simulink model "PalletizeBoxesUsingCobot"  (R2024b)
settings: Solver=FixedStepDiscrete  StartTime=0.0  StopTime=Inf  FixedStep=0.01  RelTol=1e-3
PreLoadFcn:
  | rbt = exampleHelperSetUpCobot();
  | 
  | %maxNumOfBoxes = 30;
  | %boxDim = 0.2;
  | boxPosition = [-0.65 0.45 0.6];
  | 
  | % initSim.m
  | boxData = readmatrix('boxDimensions.xlsx');  % Now it's a double matrix
  | assignin('base', 'boxData', boxData);
InitFcn:
  | goal_data = readmatrix('rectangle_placements_ROT.xlsx');
StartFcn:
  | coder.extrinsic("spawnBox")
  | 
  | % Spawn the first box on the bench
  | K = [0.2, 0.2, 0.2];
  | spawnBox(0,boxPosition,K)
values from neighbouring files (symbols this model uses):
  boxDim = 0.2    [Rbt_setup.m]
  maxNumOfBoxes = 30    [Rbt_setup.m]
undefined symbols (not defined in the file or in its folder): A2, A20, I12, N2, N20, O12, O2
libraries: robotcorelib x3, robotmaniplib x3, sim3dlib x2, robotsim3dlib x1, simulink x1
settings Model: SimulationMode=accelerator  PauseTimes=1  Creator=araman  LastModifiedBy=admin
settings DebuggingCC: ReadBeforeWriteMsg=DisableAll  WriteAfterWriteMsg=DisableAll  WriteAfterReadMsg=DisableAll  MultiTaskDSMMsg=none
settings ModelReferenceCC: UpdateModelReferenceTargets=IfOutOfDate
settings SFSimCC: SFSimEcho=off

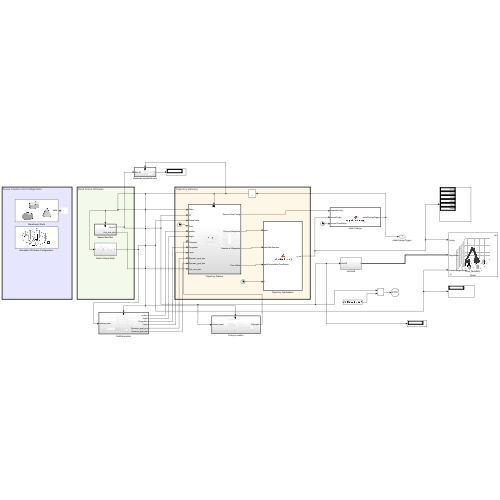
[thumbnail: Simulink's stored preview of the top-level diagram]
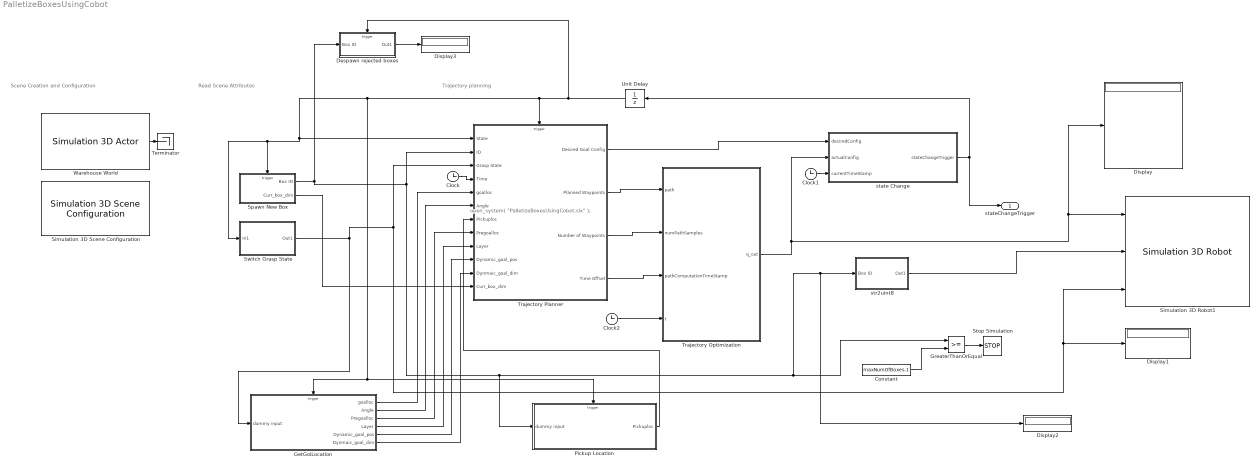
== system PalletizeBoxesUsingCobot ==
  note: open_system( "PalletizeBoxesUsingCobot.slx" );
  note: Trajectory planning
  note: Scene Creation and Configuration
  note: Read Scene Attributes
  Clock : Clock
  Clock1 : Clock
  Clock2 : Clock
  Constant : Constant  Value=maxNumOfBoxes-1
  Despawn rejected boxes : Subsystem  TreatAsAtomicUnit=on
  Display{,1..3} (4 alike) : Display
  GetGolLocation : Subsystem
  GreaterThanOrEqual : RelationalOperator  OutDataTypeStr=boolean  RndMeth=Simplest  InputSameDT=off
  Pickup Location : Subsystem  TreatAsAtomicUnit=on
  Simulation 3D Robot1 : robotsim3dlib/Simulation 3D Robot  actorInputType=RigidBodyTree Object  RigidBodyTree=rbt  ActorName=Robot  existActorChekBox=off  initialTrans=[0 0 0]  initialRot=[0 0 0]  initialConfig=[2.852 -1.623 2.216 4.223 -1.558 4.379]  EndEffector=4cup_assembly  eeOffsetInpChekBox=off  eeTargetTrans=[0 -0.2 0]  eeTargetRot=[0 0 0]  enableRegionGraspChekBox=off  regionGraspInpChekBox=off  eeTargTransDiff=[0.2 0.2 0.2]  eeTargRotDiff=[0 0 0]  inpConfEnbVal=on  inpGraspEnbVal=on  inpTransEnbVal=off  outConfEnbVal=off  outGraspEnbVal=off  outTransEnbVal=off  SampleTime=-1  ActorType=SimulinkVehicle  ID=C  aMode=6  ActorTag=Robot  Mesh=RigidBodyTree
  "Simulation 3D Scene Configuration " : sim3dlib/Simulation 3D Scene Configuration  Priority=0  ProjectFormat=Default Scenes  SceneDesc=Empty scene  ProjectName=C:\Program Files\MATLAB\R2024b\toolbox\shared\sim3d_projects\automotive_project_windows\UE\WindowsNoEditor\VehicleSimulation.exe  ScenePath=/Game/Maps/EmptyScene  EnableOpenDRIVE=off  vehTagList={'Custom';'Robot';'Scene Origin';'Warehouse'}  vehTag=Robot  FreeCameraInitialTranslation=[0, 0, 5]  FreeCameraDefaultInitialTranslation=[-6, 0, 2]  FreeCameraInitialRotation=[0, -90, 0]  FreeCameraDefaultInitialRotation=[0, -15, 0]  OpVisEn=off  Ts=0.02  EnableWindow=on  EnableRemoteAccess=off  EnableWeather=off  SunAzimuth=90  SunAltitude=40.0  EnableGeospatialSun=off  Latitude=0  Longitude=0  Date=2023-01-01  Time=10:30:00  GeoTimeZone=-5.0  SunDaylightSaving=off  wind=1  clouds=10  EnableVolumetricClouds=off  CloudCoverage=0  CloudAltitude=6  fog=0  rain=0  RaindropsEffect=off  SnowDensity=0  EnableGeospatial=off  UseTrueOrigin=off  OriginHeight=200  OriginLatitude=40.744652  OriginLongitude=-73.988864  MapStyle=Aerial  AdditionalAssetIDs=[]  UseAdvancedSunSky=off  SolarTime=11  TimeZone=-5  Day=21  Month=9  Year=2022  UseDaylightSavingTime=on  DSTStartDay=10  DSTStartMonth=3  DSTEndDay=3  DSTEndMonth=11  DSTSwitchHour=2  sensorTag=MainCamera2  sensorId=2  sensorName=MainCamera2  mountLoc=Origin  offsetFlag=off  tmountOffset=[0, 0, 0]  rmountOffset=[0, 0, 0]  HorizontalResolution=1280  VerticalResolution=720  HorizontalFOV=60  mountPoint=[0 0 0]  mountOrientation=[0 0 0]  aMode=6  ID=2  GeoTrigger=Inactive
      settings: LibrarySourceBlock=robotsim3dlib/Simulation 3D Scene Configuration
  Spawn New Box : Subsystem  TreatAsAtomicUnit=on
  Stop Simulation : Stop
  Switch Grasp State : Subsystem
  Terminator : Terminator
  Trajectory Optimization : MATLAB Function  TreatAsAtomicUnit=on
  Trajectory Planner : Subsystem
  Unit Delay : UnitDelay  InitialCondition=-1  SampleTime=-1  HasFrameUpgradeWarning=on
  Warehouse World : sim3dlib/Simulation 3D Actor  Priority=1  ActorName=Warehouse  ParentName=Scene Origin  Operation=Create at setup  InitScriptText=|  SampleTime=-1  Translation=single([0 0 0])  Rotation=single([0 0 0])  Scale=single([1 1 1])  aMode=5  ActorTag=Warehouse  ActorType=Sim3dActor  ID=2
      | Plane = sim3d.Actor(ActorName='Plane');
      | Plane.createShape('plane',[5 6 0.1]);
      | Plane.PreciseContacts = true;
      | Plane.Color = [81, 94, 120]/256;
      | add(World,Plane,Actor);
      | 
      | Base = sim3d.Actor('ActorName','collBase');
      | Base.createShape('box',[0.25,0.25,0.5]);
      | Base.Translation = [0,0.1,0.25];
      | Base.Color = [87, 67, 60]/256;
      | add(World,Base,Actor);
      | 
      | %Box spawn bench
      | Bench = sim3d.Actor('ActorName','collBench');
      | Bench.createShape('box',[0.8 0.8 0.5]);
      | Bench.Translation = [-0.5 -0.7 0.25];
      | Bench.Color = [87, 67, 60]/256;
      | add(World,Bench,Actor);
      | 
      | %Rejection conveyer
      | Bench_R = sim3d.Actor('ActorName','collBench_R');
      | Bench_R.createShape('box',[0.4 0.8 0.3]);
      | Bench_R.Translation = [-1.2 -0.7 0.25];
      | Bench_R.Color = [180, 40, 36]/256;
      | add(World,Bench_R,Actor);
      | 
      | 
      | %Layer 2 storage bench
      | Bench_2 = sim3d.Actor('ActorName','collBench_2');
      | Bench_2.createShape('box',[1.2 0.8 0.5]);
      | Bench_2.Translation = [0.4 0.8 0.25];
      | Bench_2.Color = [40, 170, 46]/256;
      | add(World,Bench_2,Actor);
      | 
      | 
      | Pallet = sim3d.Actor(ActorName='collPallet');
      | add(World,Pallet,Actor)
      | load(Pallet,"SceneAssets/PalletEuro.stl",0.001*[1 1 1]);
      | Pallet.Translation = [-1.1 -0.1 0];
  state Change : MATLAB Function  TreatAsAtomicUnit=on
  str2uint8 : Subsystem
  stateChangeTrigger : Outport
  wires:
  Warehouse World/1 -> Terminator/1
  Unit Delay/1 -> GetGolLocation/Trigger, Pickup Location/Trigger, Spawn New Box/Trigger, Switch Grasp State/1(In1), Trajectory Planner/1(State), Trajectory Planner/Trigger, Despawn rejected boxes/Trigger
  Clock/1 -> Trajectory Planner/4(Time)
  Trajectory Planner/2(Planned Waypoints) -> Trajectory Optimization/1(path)
  Trajectory Planner/3(Number of Waypoints) -> Trajectory Optimization/2(numPathSamples)
  Trajectory Planner/4(Time Offset) -> Trajectory Optimization/3(pathComputationTimeStamp)
  Trajectory Planner/1(Desired Goal Config) -> state Change/1(desiredConfig)
  Spawn New Box/1(Box ID) -> Pickup Location/1(dummy input), Display2/1, str2uint8/1(Box ID), GreaterThanOrEqual/1, Trajectory Planner/2(ID), Despawn rejected boxes/1(Box ID)
  Clock1/1 -> state Change/3(currentTimeStamp)
  state Change/1(stateChangeTrigger) -> stateChangeTrigger/1, Unit Delay/1
  Clock2/1 -> Trajectory Optimization/4(t)
  Switch Grasp State/1(Out1) -> Simulation 3D Robot1/3, Display1/1, Trajectory Planner/3(Grasp State), GetGolLocation/1(dummy input)
  Trajectory Optimization/1(q_out) -> state Change/2(actualConfig), Display/1, Simulation 3D Robot1/1
  Constant/1 -> GreaterThanOrEqual/2
  GreaterThanOrEqual/1 -> Stop Simulation/1
  GetGolLocation/1(goalloc) -> Trajectory Planner/5(goalloc)
  GetGolLocation/2(Angle) -> Trajectory Planner/6(Angle)
  str2uint8/1(Out1) -> Simulation 3D Robot1/2
  Pickup Location/1(Pickuploc) -> Trajectory Planner/7(Pickuploc)
  GetGolLocation/3(Pregoalloc) -> Trajectory Planner/8(Pregoalloc)
  GetGolLocation/4(Layer) -> Trajectory Planner/9(Layer)
  Despawn rejected boxes/1(Out1) -> Display3/1
  GetGolLocation/5(Dynamic_goal_pos) -> Trajectory Planner/10(Dynamic_goal_pos)
  GetGolLocation/6(Dynmaic_goal_dim) -> Trajectory Planner/11(Dynmaic_goal_dim)
  Spawn New Box/2(Curr_box_dim) -> Trajectory Planner/12(Curr_box_dim)

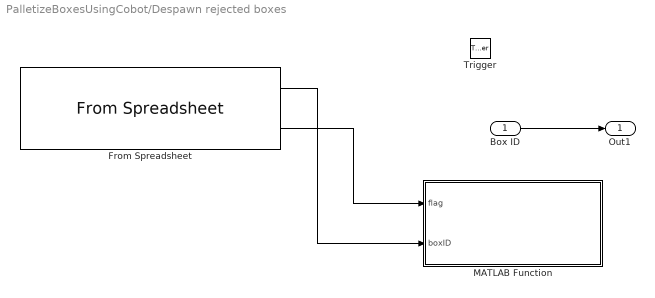
== system PalletizeBoxesUsingCobot/Despawn rejected boxes ==
  Box ID : Inport
  Trigger : TriggerPort  VariantControl=(inherit)
  From Spreadsheet : FromSpreadsheet  FileName=box_pick_goal_schedule_1.xlsx  Range=A2:A20,N2:N20  TreatFirstColumnAs=Data  SampleTime=-1
  MATLAB Function : MATLAB Function  TreatAsAtomicUnit=on
  Out1 : Outport
  wires:
  Box ID/1 -> Out1/1
  From Spreadsheet/2 -> MATLAB Function/1(flag)
  From Spreadsheet/1 -> MATLAB Function/2(boxID)

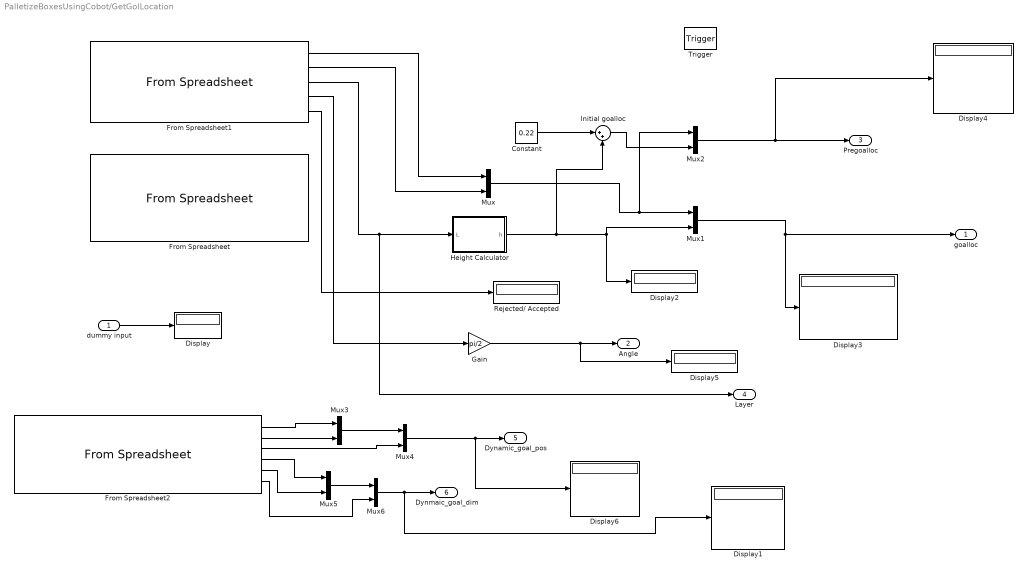
== system PalletizeBoxesUsingCobot/GetGolLocation ==
  dummy input : Inport
  Trigger : TriggerPort  VariantControl=(inherit)  PortDimensions=1
  Constant : Constant  Value=0.22
  Display{,1..6} (7 alike) : Display
  From Spreadsheet : FromSpreadsheet  FileName=test.xlsx  SheetName=Sheet3  Range=A2:B8, G2:H8, I2:I8  TreatFirstColumnAs=Data  SampleTime=-1
  From Spreadsheet1 : FromSpreadsheet  FileName=box_pick_goal_schedule_14.xlsx  SheetName=Sheet2  Range=E2:F11, K2:K11, L2:L11, N2:N11  TreatFirstColumnAs=Data  SampleTime=-1
  From Spreadsheet2 : FromSpreadsheet  FileName=box_pick_goal_schedule_14.xlsx  SheetName=Sheet3  Range=E2:I12,O2:O12  TreatFirstColumnAs=Data  SampleTime=-1
  Gain : Gain  Gain=pi/2
  Height Calculator : MATLAB Function  TreatAsAtomicUnit=on
  Initial goalloc : Sum  Inputs=|++
  Mux{,1..6} (7 alike) : Mux  Inputs=2
  Rejected/ Accepted : Display
  goalloc : Outport
  Angle : Outport  Port=2
  Pregoalloc : Outport  Port=3
  Layer : Outport  Port=4
  Dynamic_goal_pos : Outport  Port=5
  Dynmaic_goal_dim : Outport  Port=6
  wires:
  Mux/1 -> Mux1/1, Mux2/1
  dummy input/1 -> Display/1
  Mux1/1 -> Display3/1, goalloc/1
  Gain/1 -> Display5/1, Angle/1
  Height Calculator/1(h) -> Mux1/2, Display2/1, Initial goalloc/2
  Constant/1 -> Initial goalloc/1
  Initial goalloc/1 -> Mux2/2
  Mux2/1 -> Display4/1, Pregoalloc/1
  From Spreadsheet1/3 -> Layer/1, Height Calculator/1(L)
  From Spreadsheet1/2 -> Mux/2
  From Spreadsheet1/1 -> Mux/1
  From Spreadsheet1/4 -> Gain/1
  From Spreadsheet1/5 -> Rejected/ Accepted/1
  From Spreadsheet2/1 -> Mux3/1
  From Spreadsheet2/2 -> Mux3/2
  Mux3/1 -> Mux4/1
  From Spreadsheet2/3 -> Mux4/2
  From Spreadsheet2/4 -> Mux5/1
  From Spreadsheet2/5 -> Mux5/2
  Mux5/1 -> Mux6/1
  From Spreadsheet2/6 -> Mux6/2
  Mux4/1 -> Display6/1, Dynamic_goal_pos/1
  Mux6/1 -> Display1/1, Dynmaic_goal_dim/1

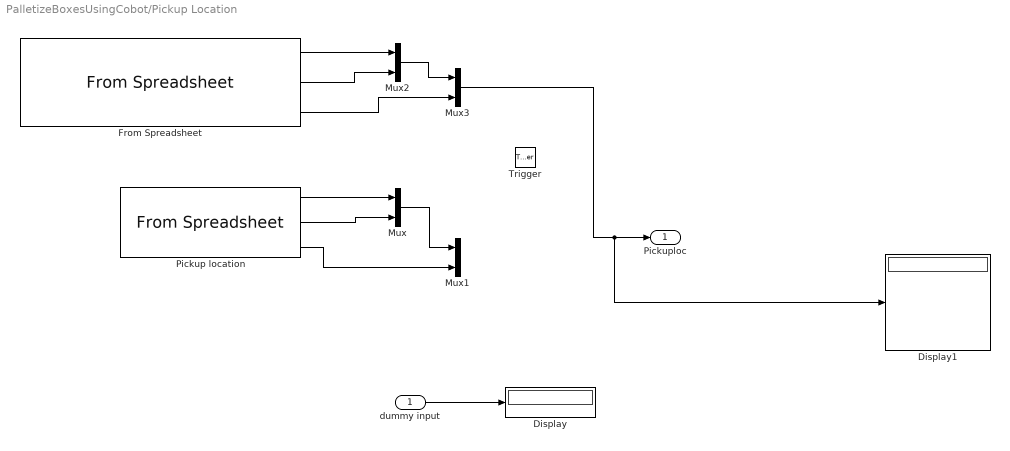
== system PalletizeBoxesUsingCobot/Pickup Location ==
  dummy input : Inport
  Trigger : TriggerPort  TriggerType=falling  VariantControl=(inherit)
  Display : Display
  Display1 : Display
  From Spreadsheet : FromSpreadsheet  FileName=box_pick_goal_schedule_14.xlsx  SheetName=Sheet2  Range=B2:D10  TreatFirstColumnAs=Data  SampleTime=-1
  Mux{,1..3} (4 alike) : Mux  Inputs=2
  Pickup location : FromSpreadsheet  FileName=test.xlsx  SheetName=Sheet3  Range=J2:L8  TreatFirstColumnAs=Data  SampleTime=-1
  Pickuploc : Outport
  wires:
  Pickup location/1 -> Mux/1
  Pickup location/2 -> Mux/2
  Pickup location/3 -> Mux1/2
  Mux/1 -> Mux1/1
  dummy input/1 -> Display/1
  From Spreadsheet/1 -> Mux2/1
  From Spreadsheet/2 -> Mux2/2
  Mux2/1 -> Mux3/1
  From Spreadsheet/3 -> Mux3/2
  Mux3/1 -> Display1/1, Pickuploc/1

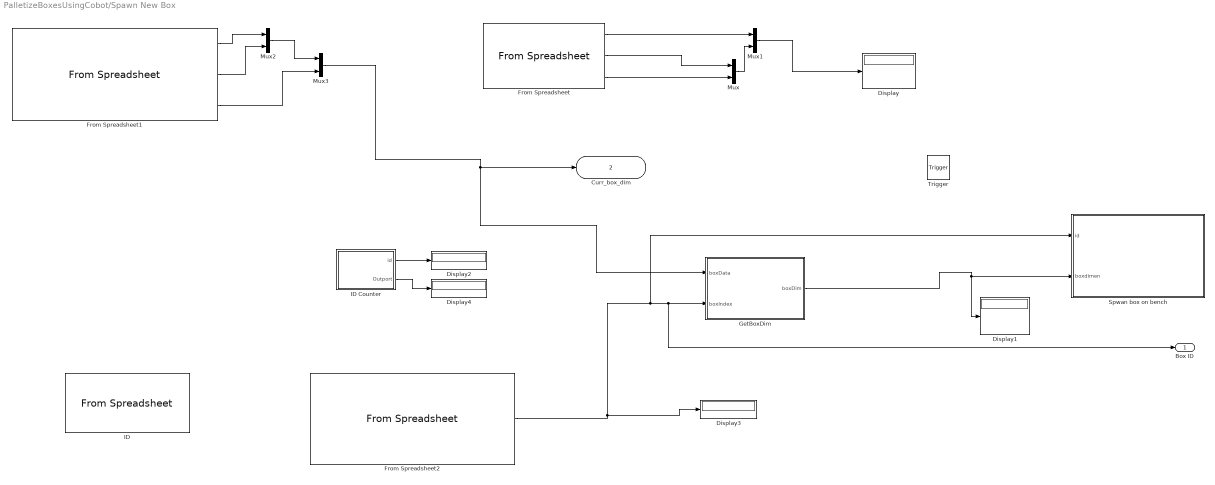
== system PalletizeBoxesUsingCobot/Spawn New Box ==
  Trigger : TriggerPort  TriggerType=falling  VariantControl=(inherit)
  Display{,1..4} (5 alike) : Display
  From Spreadsheet : FromSpreadsheet  FileName=test.xlsx  SheetName=Sheet4  Range=B2:C5, E2:E5  OutDataTypeStr=double  TreatFirstColumnAs=Data  SampleTime=-1  OutputAfterLastPoint=Ground value
  From Spreadsheet1 : FromSpreadsheet  FileName=Boxes.xlsx  SheetName=Sheet2  Range=B2:C8, E2:E8  TreatFirstColumnAs=Data  SampleTime=-1  OutputAfterLastPoint=Ground value
  From Spreadsheet2 : FromSpreadsheet  FileName=box_pick_goal_schedule_14.xlsx  SheetName=Sheet2  Range=A2:A10  TreatFirstColumnAs=Data  SampleTime=-1  OutputAfterLastPoint=Ground value
  GetBoxDim : MATLAB Function  TreatAsAtomicUnit=on
  ID : FromSpreadsheet  FileName=test.xlsx  SheetName=Sheet3  Range=N2:N8  TreatFirstColumnAs=Data  SampleTime=-1
  ID Counter : Subsystem
  Mux{,1..3} (4 alike) : Mux  Inputs=2
  Spwan box on bench : MATLAB Function  TreatAsAtomicUnit=on
  Box ID : Outport
  Curr_box_dim : Outport  Port=2
  wires:
  GetBoxDim/1(boxDim) -> Display1/1, Spwan box on bench/2(boxdimen)
  From Spreadsheet/2 -> Mux/1
  From Spreadsheet/3 -> Mux/2
  From Spreadsheet/1 -> Mux1/1
  Mux/1 -> Mux1/2
  ID Counter/1(id) -> Display2/1
  ID Counter/2(Outport) -> Display4/1
  Mux1/1 -> Display/1
  From Spreadsheet1/1 -> Mux2/1
  From Spreadsheet1/2 -> Mux2/2
  Mux2/1 -> Mux3/1
  From Spreadsheet1/3 -> Mux3/2
  Mux3/1 -> GetBoxDim/1(boxData), Curr_box_dim/1
  From Spreadsheet2/1 -> Display3/1, Spwan box on bench/1(id), Box ID/1, GetBoxDim/2(boxIndex)

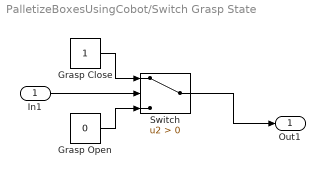
== system PalletizeBoxesUsingCobot/Switch Grasp State ==
  In1 : Inport
  Grasp Close : Constant  OutDataTypeStr=boolean
  Grasp Open : Constant  Value=0  OutDataTypeStr=boolean
  Switch : Switch  Criteria=u2 > Threshold  SaturateOnIntegerOverflow=off  InputSameDT=off
  Out1 : Outport
  wires:
  Grasp Close/1 -> Switch/1
  Switch/1 -> Out1/1
  Grasp Open/1 -> Switch/3
  In1/1 -> Switch/2

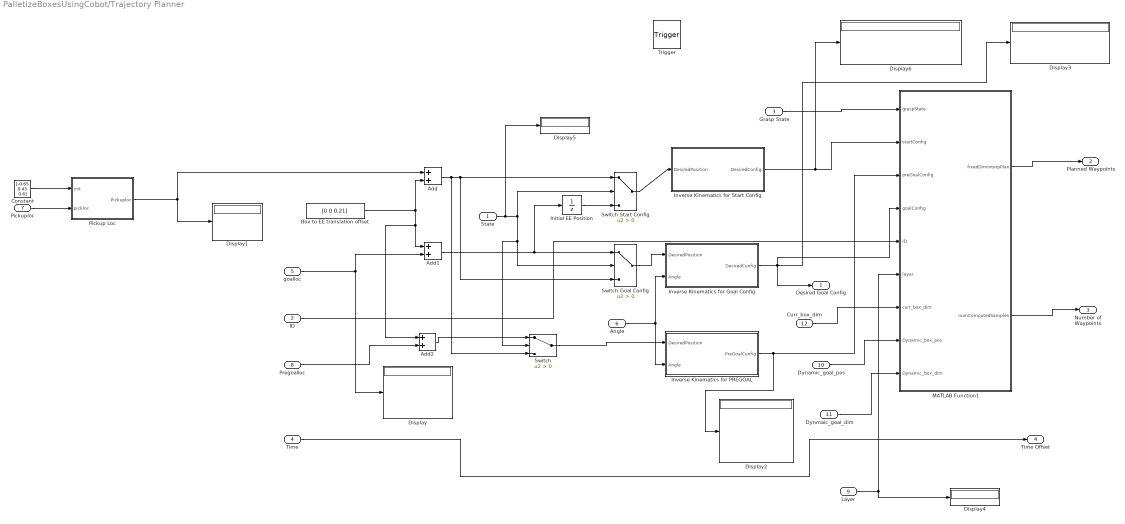
== system PalletizeBoxesUsingCobot/Trajectory Planner ==
  State : Inport
  ID : Inport  Port=2
  Grasp State : Inport  Port=3
  Time : Inport  Port=4
  goalloc : Inport  Port=5
  Angle : Inport  Port=6
  Pickuploc : Inport  Port=7
  Pregoalloc : Inport  Port=8
  Layer : Inport  Port=9
  Dynamic_goal_pos : Inport  Port=10
  Dynmaic_goal_dim : Inport  Port=11
  Curr_box_dim : Inport  Port=12
  Trigger : TriggerPort  TriggerType=either  VariantControl=(inherit)  OutputDataType=double  InitialTriggerSignalState=zero  PortDimensions=1
  Add : Sum
  Add1 : Sum
  Add2 : Sum
  Box to EE translation offset : Constant  Value=[0 0 0.21]  VectorParams1D=off
  Constant : Constant  Value=[-0.65 0.45 0.6]
  Display{,1..6} (7 alike) : Display
  Initial EE Position : UnitDelay  InitialCondition=[-0.6 0 0.8]  SampleTime=-1  HasFrameUpgradeWarning=on
  Inverse Kinematics for Goal Config : Subsystem
  Inverse Kinematics for PREGOAL : Subsystem
  Inverse Kinematics for Start Config : Subsystem
  MATLAB Function1 : MATLAB Function  TreatAsAtomicUnit=on
  Pickup Loc : MATLAB Function  TreatAsAtomicUnit=on
  Switch : Switch  Criteria=u2 > Threshold  SaturateOnIntegerOverflow=off  InputSameDT=off
  Switch Goal Config : Switch  Criteria=u2 > Threshold  SaturateOnIntegerOverflow=off  InputSameDT=off
  Switch Start Config : Switch  Criteria=u2 > Threshold  SaturateOnIntegerOverflow=off  InputSameDT=off
  Desired Goal Config : Outport
  Planned Waypoints : Outport  Port=2
  Number of Waypoints : Outport  Port=3
  Time Offset : Outport  Port=4
  wires:
  Time/1 -> Time Offset/1
  Switch Start Config/1 -> Inverse Kinematics for Start Config/1(DesiredPosition)
  Initial EE Position/1 -> Switch Start Config/3
  Switch Goal Config/1 -> Inverse Kinematics for Goal Config/1(DesiredPosition)
  Add/1 -> Switch/3, Switch Start Config/1, Switch Goal Config/3
  State/1 -> Display5/1, Switch Start Config/2, Switch Goal Config/2, Switch/2
  Add1/1 -> Initial EE Position/1, Switch Goal Config/1
  goalloc/1 -> Display/1, Add1/2
  Angle/1 -> Inverse Kinematics for Goal Config/2(Angle), Inverse Kinematics for PREGOAL/2(Angle)
  Pickuploc/1 -> Pickup Loc/2(pickloc)
  Constant/1 -> Pickup Loc/1(init)
  Pickup Loc/1(Pickuploc) -> Display1/1, Add/1
  Inverse Kinematics for PREGOAL/1(PreGoalConfig) -> MATLAB Function1/3(preGoalConfig), Display2/1
  Pregoalloc/1 -> Add2/2
  Box to EE translation offset/1 -> Add/2, Add1/1, Add2/1
  Add2/1 -> Switch/1
  Switch/1 -> Inverse Kinematics for PREGOAL/1(DesiredPosition)
  Inverse Kinematics for Goal Config/1(DesiredConfig) -> Display3/1, Desired Goal Config/1, MATLAB Function1/4(goalConfig)
  MATLAB Function1/1(fixedDimInterpPlan) -> Planned Waypoints/1
  MATLAB Function1/2(numComputedSamples) -> Number of Waypoints/1
  Grasp State/1 -> MATLAB Function1/1(graspState)
  Inverse Kinematics for Start Config/1(DesiredConfig) -> Display6/1, MATLAB Function1/2(startConfig)
  ID/1 -> MATLAB Function1/5(ID)
  Layer/1 -> MATLAB Function1/6(layer), Display4/1
  Dynmaic_goal_dim/1 -> MATLAB Function1/9(Dynamic_box_dim)
  Dynamic_goal_pos/1 -> MATLAB Function1/8(Dynamic_box_pos)
  Curr_box_dim/1 -> MATLAB Function1/7(curr_box_dim)

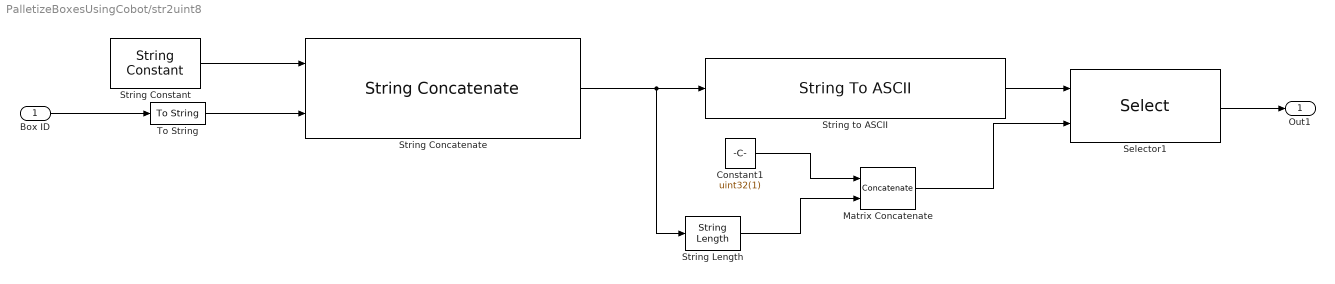
== system PalletizeBoxesUsingCobot/str2uint8 ==
  Box ID : Inport
  Constant1 : Constant  Value=uint32(1)
  Matrix Concatenate : Concatenate  ConcatenateDimension=2
  Selector1 : Selector  InputPortWidth=12  IndexOptions=Starting and ending indices (port)  Indices=[1 3]  OutputSizes=1
  String Concatenate : StringConcatenate
  String Constant : StringConstant  String="\"collBox\""
  String Length : StringLength
  String to ASCII : StringToASCII  OutputVectorSize=12
  To String : ToString
  Out1 : Outport
  wires:
  String Constant/1 -> String Concatenate/1
  Constant1/1 -> Matrix Concatenate/1
  String Length/1 -> Matrix Concatenate/2
  String Concatenate/1 -> String Length/1, String to ASCII/1
  Box ID/1 -> To String/1
  Matrix Concatenate/1 -> Selector1/2
  String to ASCII/1 -> Selector1/1
  To String/1 -> String Concatenate/2
  Selector1/1 -> Out1/1

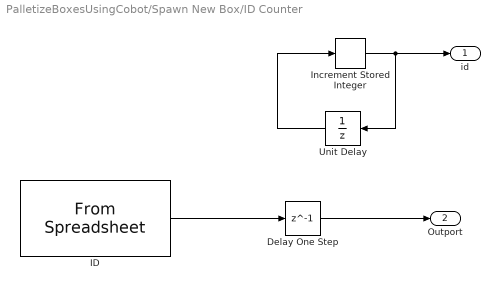
== system PalletizeBoxesUsingCobot/Spawn New Box/ID Counter ==
  Delay One Step : Delay  DelayLength=1
  ID : FromSpreadsheet  FileName=test.xlsx  SheetName=Sheet3  Range=M2:M7  TreatFirstColumnAs=Data  SampleTime=-1
  Increment Stored Integer : simulink/Additional Math & Discrete/Additional Math: Increment - Decrement/Increment Stored Integer
  Unit Delay : UnitDelay  SampleTime=-1  HasFrameUpgradeWarning=on
  id : Outport
  Outport : Outport  Port=2
  wires:
  Increment Stored Integer/1 -> id/1, Unit Delay/1
  Unit Delay/1 -> Increment Stored Integer/1
  ID/1 -> Delay One Step/1
  Delay One Step/1 -> Outport/1

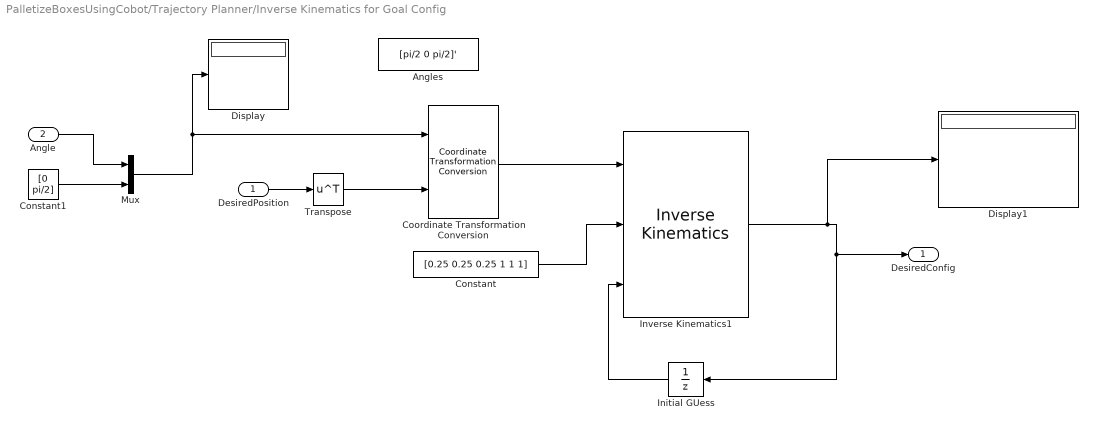
== system PalletizeBoxesUsingCobot/Trajectory Planner/Inverse Kinematics for Goal Config ==
  DesiredPosition : Inport
  Angle : Inport  Port=2
  Angles : Constant  Value=[pi/2 0 pi/2]'  VectorParams1D=off
  Constant : Constant  Value=[0.25 0.25 0.25 1 1 1]
  Constant1 : Constant  Value=[0 pi/2]
  Coordinate Transformation Conversion : robotcorelib/Coordinate Transformation Conversion  InputRepresentation=Euler Angles  InputEulerSequence=ZYX  ShowTrVecInputPort=on  OutputRepresentation=Homogeneous Transformation  OutputEulerSequence=ZYX  ShowTrVecOutputPort=on  SimulateUsing=Interpreted execution
  Display : Display
  Display1 : Display
  Initial GUess : UnitDelay  InitialCondition="[2.8471   -1.6598    2.1329    4.2393   -1.5708    4.4179]'"  SampleTime=-1  HasFrameUpgradeWarning=on
  Inverse Kinematics1 : robotmaniplib/Inverse Kinematics  RigidBodyTree=rbt  EndEffector=4cup_assembly  ShowInfo=off  SolverName=BFGS Gradient Projection  EnforceJointLimits=on  MaxIterations=40  MaxTime=10  GradientTolerance=1e-7  SolutionTolerance=1e-6  StepTolerance=1e-14  ErrorChangeTolerance=1e-12  UseErrorDamping=on  DampingBias=0.0025  SimulateUsing=Code generation
  Mux : Mux  Inputs=2
  Transpose : Math  Operator=transpose
  DesiredConfig : Outport
  wires:
  Constant/1 -> Inverse Kinematics1/2
  Coordinate Transformation Conversion/1 -> Inverse Kinematics1/1
  DesiredPosition/1 -> Transpose/1
  Initial GUess/1 -> Inverse Kinematics1/3
  Inverse Kinematics1/1 -> Display1/1, Initial GUess/1, DesiredConfig/1
  Transpose/1 -> Coordinate Transformation Conversion/2
  Constant1/1 -> Mux/2
  Mux/1 -> Display/1, Coordinate Transformation Conversion/1
  Angle/1 -> Mux/1

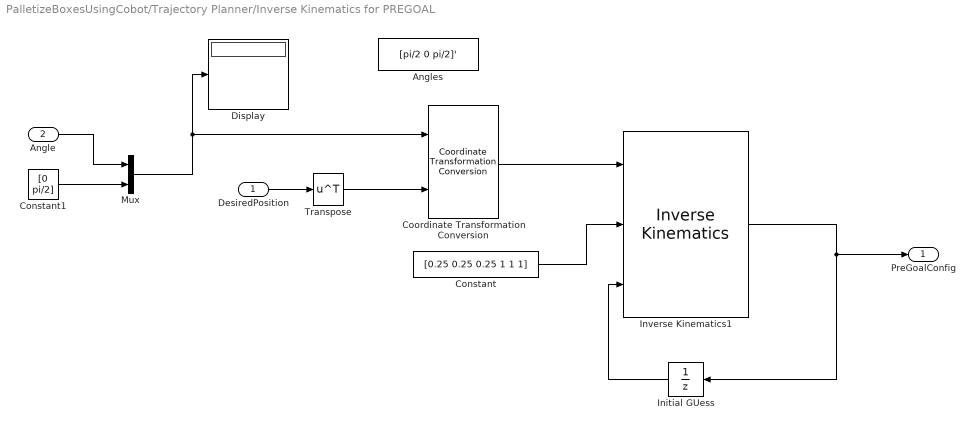
== system PalletizeBoxesUsingCobot/Trajectory Planner/Inverse Kinematics for PREGOAL ==
  DesiredPosition : Inport
  Angle : Inport  Port=2
  Angles : Constant  Value=[pi/2 0 pi/2]'  VectorParams1D=off
  Constant : Constant  Value=[0.25 0.25 0.25 1 1 1]
  Constant1 : Constant  Value=[0 pi/2]
  Coordinate Transformation Conversion : robotcorelib/Coordinate Transformation Conversion  InputRepresentation=Euler Angles  InputEulerSequence=ZYX  ShowTrVecInputPort=on  OutputRepresentation=Homogeneous Transformation  OutputEulerSequence=ZYX  ShowTrVecOutputPort=on  SimulateUsing=Interpreted execution
  Display : Display
  Initial GUess : UnitDelay  InitialCondition="[2.8471   -1.6598    2.1329    4.2393   -1.5708    4.4179]'"  SampleTime=-1  HasFrameUpgradeWarning=on
  Inverse Kinematics1 : robotmaniplib/Inverse Kinematics  RigidBodyTree=rbt  EndEffector=4cup_assembly  ShowInfo=off  SolverName=BFGS Gradient Projection  EnforceJointLimits=on  MaxIterations=40  MaxTime=10  GradientTolerance=1e-7  SolutionTolerance=1e-6  StepTolerance=1e-14  ErrorChangeTolerance=1e-12  UseErrorDamping=on  DampingBias=0.0025  SimulateUsing=Code generation
  Mux : Mux  Inputs=2
  Transpose : Math  Operator=transpose
  PreGoalConfig : Outport
  wires:
  Constant/1 -> Inverse Kinematics1/2
  Coordinate Transformation Conversion/1 -> Inverse Kinematics1/1
  DesiredPosition/1 -> Transpose/1
  Initial GUess/1 -> Inverse Kinematics1/3
  Inverse Kinematics1/1 -> Initial GUess/1, PreGoalConfig/1
  Transpose/1 -> Coordinate Transformation Conversion/2
  Constant1/1 -> Mux/2
  Mux/1 -> Display/1, Coordinate Transformation Conversion/1
  Angle/1 -> Mux/1

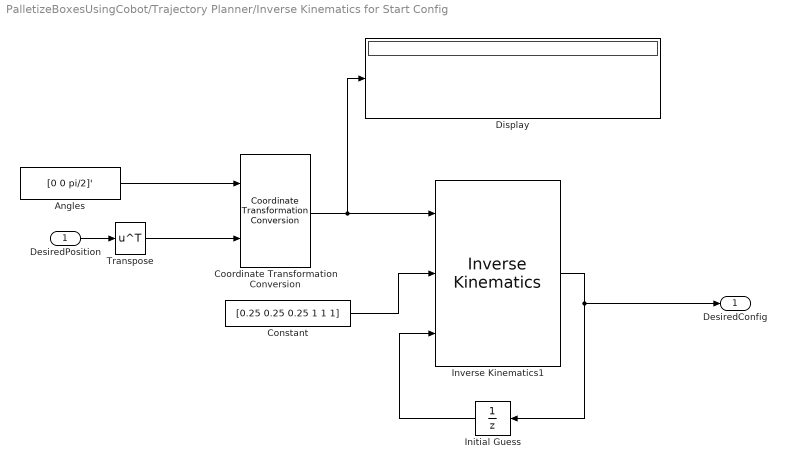
== system PalletizeBoxesUsingCobot/Trajectory Planner/Inverse Kinematics for Start Config ==
  DesiredPosition : Inport
  Angles : Constant  Value=[0 0 pi/2]'  VectorParams1D=off
  Constant : Constant  Value=[0.25 0.25 0.25 1 1 1]
  Coordinate Transformation Conversion : robotcorelib/Coordinate Transformation Conversion  InputRepresentation=Euler Angles  InputEulerSequence=ZYX  ShowTrVecInputPort=on  OutputRepresentation=Homogeneous Transformation  OutputEulerSequence=ZYX  ShowTrVecOutputPort=on  SimulateUsing=Interpreted execution
  Display : Display
  Initial Guess : UnitDelay  InitialCondition="[-0.0724   -0.8022    1.6836    3.8   -1.5708    1.3514]'"  SampleTime=-1  HasFrameUpgradeWarning=on
  Inverse Kinematics1 : robotmaniplib/Inverse Kinematics  RigidBodyTree=rbt  EndEffector=4cup_assembly  ShowInfo=off  SolverName=BFGS Gradient Projection  EnforceJointLimits=on  MaxIterations=40  MaxTime=10  GradientTolerance=1e-7  SolutionTolerance=1e-6  StepTolerance=1e-14  ErrorChangeTolerance=1e-12  UseErrorDamping=on  DampingBias=0.0025  SimulateUsing=Code generation
  Transpose : Math  Operator=transpose
  DesiredConfig : Outport
  wires:
  Constant/1 -> Inverse Kinematics1/2
  Angles/1 -> Coordinate Transformation Conversion/1
  Inverse Kinematics1/1 -> DesiredConfig/1, Initial Guess/1
  Initial Guess/1 -> Inverse Kinematics1/3
  Coordinate Transformation Conversion/1 -> Display/1, Inverse Kinematics1/1
  DesiredPosition/1 -> Transpose/1
  Transpose/1 -> Coordinate Transformation Conversion/2

== matlab function PalletizeBoxesUsingCobot/Despawn rejected boxes/MATLAB Function ==
  data: flag input; boxID input
function maybeDespawnBox(flag, boxID)
% MAYBEDESPAWNBOX deletes the box only if flag == 1
    coder.extrinsic("despawnBox");
    if flag == 1
        x = boxID-1;
        despawnBox(x); %Delete previous box
        disp(['Box ' boxID ' was rejected and has been removed.']);
    end

end

== matlab function PalletizeBoxesUsingCobot/state Change ==
  data: desiredConfig input; stateChangeTrigger output; actualConfig input; currentTimeStamp input
function stateChangeTrigger = triggerStateChange(desiredConfig,actualConfig, currentTimeStamp)

tol = sqrt(eps);
simTimeStep = 0.01; % discrete time step of the simulation

persistent stateChange timeAtStateChange
if isempty(stateChange)
    stateChange = -1;
    timeAtStateChange = 0;
end

% Ensure that the goal position is reached and held for at least one
% simulation time step
if sqrt(sum((desiredConfig-actualConfig).^2)) < tol && (currentTimeStamp - timeAtStateChange) > simTimeStep
    switch stateChange
        case -1 
            stateChange = 1;
        case 1
            stateChange = -1; 
    end
    timeAtStateChange = currentTimeStamp;
end

stateChangeTrigger = stateChange;

end

== matlab function PalletizeBoxesUsingCobot/GetGolLocation/Height Calculator ==
  data: L input; h output
function h = f(L)

if L == 0
    h = 0.65;

else
    h = 0.244 + (L-1)*0.2;
end

== matlab function PalletizeBoxesUsingCobot/Trajectory Optimization ==
  data: path input size=[6,200]; numPathSamples input; pathComputationTimeStamp input; t input; q_out output
function q_out = helperContopptraj(path, numPathSamples, pathComputationTimeStamp, t)

coder.extrinsic('contopptraj');
coder.extrinsic('optimoptions');
coder.extrinsic('fmincon'); 

VELLIM = repmat([-10  10], 6, 1);   % Velocity limits for trajectory
ACCELLIM = repmat([-15 15], 6, 1); % Acceleration limits for trajectory

% Store the last time at which the path was computed as a persistent
% variable. This allows the function to detect changes
persistent prevPathComputationTime qSolve tSolve
if isempty(prevPathComputationTime)
    prevPathComputationTime = -1;
end


if isempty(qSolve)
    qSolve = repmat([2.8471   -1.6598    2.1329    4.2393   -1.5708    4.4179]',1,500);
    tSolve = linspace(0,2,500);
end


if (pathComputationTimeStamp ~= prevPathComputationTime) && (numPathSamples > 0)
    qSolve = zeros(6,100);
    tSolve = linspace(0,1,100);
    
    
    % 1. Create a Time-Optimal Path Parameterization (TOPPRA) solver
   
% Sample time and total time
    numSamples = 100;
    totalTime = 2; % or any appropriate value
    tSolve = linspace(0, totalTime, numSamples);

% Compute trajectory using trapveltraj
    [qSolve, ~, ~] = trapveltraj(path(:,1:numPathSamples), numSamples);



end
%{
% Compute a time constrained trajectory with contoptraj
if (pathComputationTimeStamp ~= prevPathComputationTime) && (numPathSamples > 0)
    [qSolve,~,~,tSolve] = contopptraj(path(:,1:numPathSamples),VELLIM,ACCELLIM,NumSamples=100);
end
%}

%if (pathComputationTimeStamp ~= prevPathComputationTime) && (numPathSamples > 0)
    %qSolve(:,1:numPathSamples) = path(:,1:numPathSamples);
%end

% Compute the output at an instant in time t. Because contopptraj defines
% the time stamp relative to a clock that begins at zero, subtract the time
% stamp at computation time from the current time.
q_out = zeros(6,1);

maxTime = max(tSolve);
queryTime = t - pathComputationTimeStamp;
if queryTime == 0
    q_out(:) = qSolve(:,1);
elseif queryTime <= maxTime
    % Use linear interpolation to approximate the reference trajectory
    % inside the time range for which it is defined
    q_out(:) = interp1(tSolve,qSolve',queryTime);
else
    % After the trajectory end is reached, if no new trajectory is
    % computed, hold the last value
    q_out(:) = qSolve(:,end);
end

% Update the stored path computation time stamp
prevPathComputationTime = pathComputationTimeStamp;

end

== matlab function PalletizeBoxesUsingCobot/Spawn New Box/GetBoxDim ==
  data: boxData input; boxDim output; boxIndex input
function boxDim = getBoxDimension(boxData, boxIndex)
    % Get the box dimension from a table passed in as input
    %L = boxData(1,1);
    %W = boxData(1,2);
    %H = boxData(1,3);
    boxDim = boxData;
end

== matlab function PalletizeBoxesUsingCobot/Spawn New Box/Spwan box on bench ==
  data: id input; boxdimen input
function spawnBoxOnBench(id,boxdimen)
 boxPosition = [-0.65 0.45 0.6];
 boxDim = boxdimen;
 coder.extrinsic("spawnBox")
 spawnBox(id,boxPosition,boxDim)
end

== matlab function PalletizeBoxesUsingCobot/Trajectory Planner/Pickup Loc ==
  data: init input; pickloc input; Pickuploc output
function Pickuploc = f(init,pickloc)
    if pickloc == [0 0 0]
        Pickuploc = init.';
    else
        Pickuploc = pickloc.';
    end
end

== matlab function PalletizeBoxesUsingCobot/Trajectory Planner/MATLAB Function1 ==
  data: graspState input; startConfig input; preGoalConfig input; fixedDimInterpPlan output size=[6,200]; goalConfig input; ID input; numComputedSamples output; boxPosition parameter; boxDim parameter; maxNumOfBoxes parameter; layer input; curr_box_dim input; Dynamic_box_pos input; Dynamic_box_dim input
function [fixedDimInterpPlan,numComputedSamples] = helperPathPanning(graspState, startConfig,preGoalConfig,goalConfig,ID,boxPosition, boxDim, maxNumOfBoxes,layer, curr_box_dim,Dynamic_box_pos, Dynamic_box_dim)
fixedDimInterpPlan = zeros(6, 200);
numComputedSamples = 0;
coder.extrinsic("exampleHelperManipulatorRRT");
[fixedDimInterpPlan,numComputedSamples] = exampleHelperManipulatorRRT(graspState, startConfig,goalConfig,ID,boxPosition, boxDim, maxNumOfBoxes,curr_box_dim,Dynamic_box_pos, Dynamic_box_dim);
%(graspState, startConfig,preGoalConfig,goalConfig,ID,boxPosition, boxDim, maxNumOfBoxes,layer);

end
